simulink model "demonstrator"  (R2021a)
settings: Solver=VariableStepAuto  StartTime=0.0  StopTime=4000/3.2e6  RelTol=1e-3
values from neighbouring files (symbols this model uses):
  f_system = 64e6    (= 64000000)    [setup_demonstrator.m]
  fir_bbuf = reshape([fir_barker_13; fir_barker_13; fir_barker_13], [1, length(fir_barker_13)*3])    [setup_demonstrator.m]
  tx_data = [tx_data mbuf]    [setup_demonstrator.m]
undefined symbols (not defined in the file or in its folder): AXI4, designMultirateFIR, fsystem, Lite, xlfda_numerator
libraries: hdlBasic x533, hdlsllib x35, hdlDSPIP x21, hdlSSR x18, dspmlti4 x14, dspswit3 x8, dspsigops x5, vmcUtilities x4, hdlUtilities x4, simulink x3, dspsigattribs x2, commrandsrc3 x1
(part 4 of 10)

== system demonstrator/Transmitter/AXI-Stream Slave Interface ==
  s_tdata : Inport
  s_tvalid : Inport  Port=2
  s_tlast : Inport  Port=3
  Concat : hdlBasic/Concat  num_inputs=2  XmcBlockStatus=1  maskContainerNames=group1  block_type=concat  block_config=sysgen:Concat_config
  Constant : hdlBasic/Constant  const=0  gui_display_data_type=Fixed-point  arith_type=Unsigned  n_bits=8  bin_pt=0  preci_type=Single  exp_width=8  frac_width=24  explicit_period=off  period=1  XmcBlockStatus=1  maskContainerNames=tabcontainer1  block_type=constant  block_config=sysgen:Constant_config
  Convert : hdlBasic/Convert  gui_display_data_type=Fixed-point  arith_type=Unsigned  n_bits=1  bin_pt=0  float_type=Single  exp_bits=8  fraction_bits=24  quantization=Truncate  overflow=Wrap  en=off  latency=0  pipeline=off  XmcBlockStatus=1  maskContainerNames=group2  block_type=convert  block_config=sysgen:Convert_config
  Down Sample : hdlBasic/Down Sample  sample_ratio=128e6/12.5e3  sample_phase=First Value of Frame  en=off  rst=off  latency=0  XmcBlockStatus=1  maskContainerNames=group1  block_type=dsamp  block_config=sysgen:Downsample_config
  FIFO : hdlBasic/FIFO  mem_type=Block RAM  performance_options=Standard_FIFO  embedded_registers=off  depth=1K  use_asym_data_widths=off  asym_read_width=32  percent_nbits=2  rst=off  rst_latency=2  en=off  use_dcount=off  use_percent_full_port=off  use_almost_empty=off  almost_empty_thresh=2  use_almost_full=off  use_rd_rst_busy=off  use_wr_rst_busy=off  almost_full_thresh=1000  almost_empty_offset=[]  almost_full_offset=[]  explicit_period=off  period=[]  store_only_valid=[]  init_zero=[]  simulation_type=fast_sim  XmcBlockStatus=1  maskContainerNames=tabcontainer1  block_type=fifo  block_config=sysgen:FIFO_config
      settings: infoedit=[]
  Inverter : hdlBasic/Inverter  en=off  latency=0  XmcBlockStatus=1  maskContainerNames=group2  block_type=inv  block_config=sysgen:Inverter_config
  Inverter1 : hdlBasic/Inverter  en=off  latency=0  XmcBlockStatus=1  maskContainerNames=group2  block_type=inv  block_config=sysgen:Inverter_config
  Logical : hdlBasic/Logical  logical_function=AND  inputs=2  en=off  latency=0  precision=Full  arith_type=Unsigned  n_bits=16  bin_pt=0  align_bp=on  overflow=[]  quantization=[]  XmcBlockStatus=1  maskContainerNames=tabcontainer1  block_type=logical  block_config=sysgen:Logical_config
  Mux : hdlBasic/Mux  inputs=2  en=off  latency=0  precision=Full  arith_type=Unsigned  n_bits=16  bin_pt=14  quantization=Truncate  overflow=Wrap  XmcBlockStatus=1  maskContainerNames=tabcontainer1  block_type=mux  block_config=sysgen:Mux_config
  Register : hdlBasic/Register  init=0  rst=off  en=off  XmcBlockStatus=1  maskContainerNames=tabcontainer1  block_type=register  block_config=sysgen:Register_config
  Slice : hdlBasic/Slice  nbits=1  boolean_output=off  mode=Two Bit Locations  bit1=8  base1=LSB of Input  bit0=8  base0=LSB of Input  XmcBlockStatus=1  maskContainerNames=group1  block_type=slice  block_config=sysgen:Slice_config
  Slice1 : hdlBasic/Slice  nbits=1  boolean_output=off  mode=Two Bit Locations  bit1=7  base1=LSB of Input  bit0=0  base0=LSB of Input  XmcBlockStatus=1  maskContainerNames=group1  block_type=slice  block_config=sysgen:Slice_config
  s_axis_tdata : hdlBasic/Gateway In  gui_display_data_type=Fixed-point  arith_type=Unsigned  n_bits=8  bin_pt=0  preci_type=Single  exp_width=8  frac_width=24  rows=1  columns=1  quantization="Round  (unbiased: +/- Inf)"  overflow=Saturate  period=1/128e6  UseAsADC=off  ADCChannel='1'  interface=None  automatic_assignment=on  address_offset=hex2dec('00')  intf_name=''  intf_description=''  default_value=0  timing_constraint=None  locs_specified=off  LOCs={}  io_standard={}  inherit_from_input=off  hdl_port=on  XmcBlockStatus=1  maskContainerNames=group4  block_type=gatewayin  block_config=sysgen:gateway_in_config  block_width_w=590  block_height_w=620  block_width=640  block_height=850
  s_axis_tlast : hdlBasic/Gateway In  gui_display_data_type=Fixed-point  arith_type=Unsigned  n_bits=1  bin_pt=0  preci_type=Single  exp_width=8  frac_width=24  rows=1  columns=1  quantization="Round  (unbiased: +/- Inf)"  overflow=Saturate  period=1/128e6  UseAsADC=off  ADCChannel='1'  interface=None  automatic_assignment=on  address_offset=hex2dec('00')  intf_name=''  intf_description=''  default_value=0  timing_constraint=None  locs_specified=off  LOCs={}  io_standard={}  inherit_from_input=off  hdl_port=on  XmcBlockStatus=1  maskContainerNames=group4  block_type=gatewayin  block_config=sysgen:gateway_in_config  block_width_w=590  block_height_w=620  block_width=640  block_height=850
  s_axis_tready : hdlBasic/Gateway Out  inherit_from_input=on  hdl_port=on  rows=1  columns=1  UseAsDAC=off  DACChannel='1'  interface=None  automatic_assignment=on  address_offset=hex2dec('00')  intf_name=''  intf_description=''  timing_constraint=None  locs_specified=off  LOCs={}  io_standard={}  XmcBlockStatus=1  maskContainerNames=group4  block_type=gatewayout  block_config=sysgen:gateway_out_config  block_width_w=590  block_height_w=620  block_width=620  block_height=750
  s_axis_tvalid : hdlBasic/Gateway In  gui_display_data_type=Boolean  arith_type=Boolean  n_bits=16  bin_pt=14  preci_type=Single  exp_width=8  frac_width=24  rows=1  columns=1  quantization="Round  (unbiased: +/- Inf)"  overflow=Saturate  period=1/128e6  UseAsADC=off  ADCChannel='1'  interface=None  automatic_assignment=on  address_offset=hex2dec('00')  intf_name=''  intf_description=''  default_value=0  timing_constraint=None  locs_specified=off  LOCs={}  io_standard={}  inherit_from_input=off  hdl_port=on  XmcBlockStatus=1  maskContainerNames=group4  block_type=gatewayin  block_config=sysgen:gateway_in_config  block_width_w=590  block_height_w=620  block_width=640  block_height=850
  m_tdata : Outport  VectorParamsAs1DForOutWhenUnconnected=off
  m_tvalid : Outport  Port=2  VectorParamsAs1DForOutWhenUnconnected=off
  m_tlast : Outport  Port=3  VectorParamsAs1DForOutWhenUnconnected=off
  s_tready : Outport  Port=4  VectorParamsAs1DForOutWhenUnconnected=off
  wires:
  s_axis_tready/1 -> s_tready/1
  s_tlast/1 -> s_axis_tlast/1
  s_tvalid/1 -> s_axis_tvalid/1
  s_tdata/1 -> s_axis_tdata/1
  s_axis_tvalid/1 -> FIFO/2
  FIFO/3 -> Inverter/1
  Down Sample/1 -> Inverter1/1
  FIFO/2 -> Down Sample/1
  Register/1 -> Mux/1, Convert/1, m_tvalid/1
  Inverter/1 -> s_axis_tready/1
  Inverter1/1 -> Register/1, FIFO/3
  Logical/1 -> m_tlast/1
  Mux/1 -> m_tdata/1
  FIFO/1 -> Slice/1, Slice1/1
  Constant/1 -> Mux/2
  Convert/1 -> Logical/2
  Slice/1 -> Logical/1
  Concat/1 -> FIFO/1
  s_axis_tdata/1 -> Concat/2
  s_axis_tlast/1 -> Concat/1
  Slice1/1 -> Mux/3

== system demonstrator/Transmitter/Algorithm ==
  note: Serialize data,
      | send (pseudo-random) data from an LFSR if enabled and no input data is present
  note: Encode + pulse shape + interpolate
      | (only I component, Q is fixed at 0)
  enable_data : Inport
  enable_tx : Inport  Port=2
  s_tdata : Inport  Port=3
  s_tvalid : Inport  Port=4
  s_tlast : Inport  Port=5
  BPSK Differential Encoder : Subsystem
  BPSK LFSR : Subsystem
  Gateway Out : hdlBasic/Gateway Out  inherit_from_input=on  hdl_port=off  rows=1  columns=1  UseAsDAC=off  DACChannel='1'  interface=None  automatic_assignment=on  address_offset=hex2dec('00')  intf_name=''  intf_description=''  timing_constraint=None  locs_specified=off  LOCs={}  io_standard={}  XmcBlockStatus=1  maskContainerNames=group4  block_type=gatewayout  block_config=sysgen:gateway_out_config  block_width_w=590  block_height_w=620  block_width=620  block_height=750
  Gateway Out1 : hdlBasic/Gateway Out  inherit_from_input=on  hdl_port=off  rows=1  columns=1  UseAsDAC=off  DACChannel='1'  interface=None  automatic_assignment=on  address_offset=hex2dec('00')  intf_name=''  intf_description=''  timing_constraint=None  locs_specified=off  LOCs={}  io_standard={}  XmcBlockStatus=1  maskContainerNames=group4  block_type=gatewayout  block_config=sysgen:gateway_out_config  block_width_w=590  block_height_w=620  block_width=620  block_height=750
  Gateway Out2 : hdlBasic/Gateway Out  inherit_from_input=on  hdl_port=off  rows=1  columns=1  UseAsDAC=off  DACChannel='1'  interface=None  automatic_assignment=on  address_offset=hex2dec('00')  intf_name=''  intf_description=''  timing_constraint=None  locs_specified=off  LOCs={}  io_standard={}  XmcBlockStatus=1  maskContainerNames=group4  block_type=gatewayout  block_config=sysgen:gateway_out_config  block_width_w=590  block_height_w=620  block_width=620  block_height=750
  Interpolation : Subsystem
  RRC : Subsystem
  TX: Time Domain : Scope  NumInputPorts=3
  Terminator : Terminator
  m_tdata : Outport  VectorParamsAs1DForOutWhenUnconnected=off
  m_tvalid : Outport  Port=2  VectorParamsAs1DForOutWhenUnconnected=off
  wires:
  BPSK LFSR/1(m_tdata) -> BPSK Differential Encoder/2(s_tdata)
  BPSK Differential Encoder/1(m_tdata) -> Gateway Out/1, RRC/1(s_tdata)
  s_tlast/1 -> Terminator/1
  s_tdata/1 -> BPSK LFSR/2(s_tdata)
  s_tvalid/1 -> BPSK LFSR/3(s_tvalid)
  enable_data/1 -> BPSK LFSR/1(enable)
  RRC/1(m_tdata) -> Gateway Out2/1, Interpolation/1(s_tdata)
  Interpolation/2(m_tvalid) -> m_tvalid/1
  Interpolation/1(m_tdata) -> Gateway Out1/1, m_tdata/1
  enable_tx/1 -> BPSK Differential Encoder/1(tx_output)
  Gateway Out/1 -> TX: Time Domain/1
  Gateway Out1/1 -> TX: Time Domain/3
  Gateway Out2/1 -> TX: Time Domain/2

== system demonstrator/Transmitter/Convert Signal ==
  Data In : Inport
  Bit Slice : hdlsllib/Logic and Bit Operations/Bit Slice  lidx=15  ridx=0
      settings: SourceProductBaseCode=SL
  Bit Slice1 : hdlsllib/Logic and Bit Operations/Bit Slice  lidx=31  ridx=16
      settings: SourceProductBaseCode=SL
  Data Type Conversion : DataTypeConversion  OutDataTypeStr=fixdt(1,16,15)  ConvertRealWorld=Stored Integer (SI)
  Data Type Conversion1 : DataTypeConversion  OutDataTypeStr=fixdt(1,16,15)  ConvertRealWorld=Stored Integer (SI)
  Real-Imag to Complex : RealImagToComplex
  Data Out : Outport  VectorParamsAs1DForOutWhenUnconnected=off
  wires:
  Data Type Conversion1/1 -> Real-Imag to Complex/2
  Bit Slice/1 -> Data Type Conversion/1
  Data Type Conversion/1 -> Real-Imag to Complex/1
  Real-Imag to Complex/1 -> Data Out/1
  Data In/1 -> Bit Slice1/1, Bit Slice/1
  Bit Slice1/1 -> Data Type Conversion1/1

== system demonstrator/Transmitter/DMA Read ==
  enable : Inport
  tready : Inport  Port=2
  1-D Lookup Table : Lookup_n-D  NumberOfTableDimensions=1  BreakpointsForDimension1=[0:1:numel(tx_data)-1]  Table=tx_data  TableDataTypeStr=Inherit: Inherit from 'Table data'  ExtrapMethod=Clip  InternalRulePriority=Speed  OutDataTypeStr=Inherit: Inherit from 'Table data'  RndMeth=Simplest  InputSameDT=on
  AND : Logic  IconShape=distinctive  AllPortsSameDT=off  OutDataTypeStr=boolean
  AND1 : Logic  IconShape=distinctive  AllPortsSameDT=off  OutDataTypeStr=boolean
  Compare To Constant : simulink/Logic and Bit Operations/Compare To Constant  relop=>=  const=numel(tx_data)-1  OutDataTypeStr=boolean
  Data Type Conversion : DataTypeConversion  OutDataTypeStr=fixdt(0, ceil(log2(numel(tx_data))), 0)
  HDL Counter : hdlsllib/Sources/HDL Counter  CountType=Free running  CountInit=0  CountStep=1  CountMax=25  CountFromType=Initial value  CountFrom=0  CountResetPort=on  CountLoadPort=off  CountEnbPort=on  CountDirPort=off  CountHitOutputPort=off  CountDataType=Unsigned  CountWordLen=32  CountFracLen=0  CountSampTime=1
  Latch : Subsystem
  Rising Edge Detector : Subsystem
  tdata : Outport  VectorParamsAs1DForOutWhenUnconnected=off
  tvalid : Outport  Port=2  VectorParamsAs1DForOutWhenUnconnected=off
  tlast : Outport  Port=3  VectorParamsAs1DForOutWhenUnconnected=off
  wires:
  1-D Lookup Table/1 -> tdata/1
  Compare To Constant/1 -> AND1/1, HDL Counter/1, Latch/2(R)
  enable/1 -> Rising Edge Detector/1(Input)
  HDL Counter/1 -> Compare To Constant/1, Data Type Conversion/1
  Data Type Conversion/1 -> 1-D Lookup Table/1
  Rising Edge Detector/1(Output) -> Latch/1(S)
  AND/1 -> AND1/2, tvalid/1, HDL Counter/2
  Latch/1(Q) -> AND/2
  tready/1 -> AND/1
  AND1/1 -> tlast/1

== system demonstrator/Transmitter (SIM)/BPSK TX Generation ==
  note: Model DMA (instantiated as BD IP)
  note: Pulse shaping
  note: Input random bits in absence of data
  note: Encode symbols
  note: Scale down amplitude value to correct level
  Enable : Inport
  Bernoulli Binary Generator : commrandsrc3/Bernoulli Binary Generator  ProbabilityOfZero=0.5  SeedSource=Auto  Seed=0  SampleTime=1/100e3  SamplesPerFrame=1  OutputDataType=double  SimulateUsing=Interpreted execution
  CIC Interpolation : dspmlti4/CIC Interpolation  filtFrom=Dialog parameters  filtobj=Hm_interp  ftype=Interpolator  R=320  M=1  N=5  filterInternals=Full precision  BPS=[16 16 16 16]  FLPS=0  outputWordLength=32  outputFracLength=0  launchFVT=off  framing=Allow multirate processing  OutputFrames=off
      settings: SourceProductBaseCode=DS
  Constant : Constant  SampleTime=1/12.5e3
  DBPSK Modulator : Subsystem
  DMA Read : Subsystem
  Data Type Conversion2 : DataTypeConversion  OutDataTypeStr=fixdt(1,16,14)
  FDATool : hdlUtilities/FDATool  block_type=fdatool
      settings: infoedit=FDATool
  FIR Interpolation : dspmlti4/FIR Interpolation  FilterSource=Dialog parameters  PrivateCoeffs=0  h=xlfda_numerator('FDATool')*4  L=4  FilterObject=xlfda_numerator('FDATool')/(max(xlfda_numerator('FDATool')))  framing=Allow multirate processing  outputBufInitCond=0  roundingMode=Floor  overflowMode=off  firstCoeffMode=Binary point scaling  firstCoeffWordLength=16  firstCoeffFracLength=14  firstCoeffDataTypeStr=fixdt(1,16,14)  firstCoeffMin=[]  firstCoeffMax=[]  firstCoeffLastDataTypeStr=fixdt(1,16,14)  outputDataTypeStr=Inherit: Same as accumulator  outputMin=[]  outputMax=[]  outputLastDataTypeStr=Inherit: Same as accumulator
  Multiply : Gain  Gain=fi(0.8192, 1, 16, 14)  ParamDataTypeStr=fixdt(1,16,15)  OutDataTypeStr=fixdt(1,16,14)
  Multiport Switch : MultiPortSwitch  DataPortOrder=Zero-based contiguous  Inputs=2  zeroidx=on
  Shift Arithmetic : ArithShift  BitShiftNumber=33  BitShiftDirection=Right
  TX (SIM): Time Domain : Scope  NumInputPorts=4
  Terminator1 : Terminator
  BPSK : Outport  VectorParamsAs1DForOutWhenUnconnected=off
  wires:
  CIC Interpolation/1 -> TX (SIM): Time Domain/3, Shift Arithmetic/1
  FIR Interpolation/1 -> TX (SIM): Time Domain/2, Data Type Conversion2/1
  Bernoulli Binary Generator/1 -> Multiport Switch/2
  DMA Read/2(tvalid) -> Multiport Switch/1
  DMA Read/1(tdata) -> Multiport Switch/3
  DMA Read/3(tlast) -> Terminator1/1
  Enable/1 -> DMA Read/1(enable)
  Constant/1 -> DMA Read/2(tready)
  Multiport Switch/1 -> DBPSK Modulator/1(Input)
  Multiply/1 -> TX (SIM): Time Domain/4, BPSK/1
  DBPSK Modulator/1(Output) -> TX (SIM): Time Domain/1, FIR Interpolation/1
  Data Type Conversion2/1 -> CIC Interpolation/1
  Shift Arithmetic/1 -> Multiply/1

== system demonstrator/FINNadapter/Decimation/AXI-Stream Master Interface ==
  Re Valid In : Inport
  Re Data In : Inport  Port=2
  Im Valid In : Inport  Port=3
  Im Data In : Inport  Port=4
  Register{,1..3} (4 alike) : hdlBasic/Register  init=0  rst=off  en=off  XmcBlockStatus=1  maskContainerNames=tabcontainer1  block_type=register  block_config=sysgen:Register_config
  m_axis_im_tdata : hdlBasic/Gateway Out  inherit_from_input=off  hdl_port=on  rows=1  columns=1  UseAsDAC=off  DACChannel='1'  interface=None  automatic_assignment=on  address_offset=hex2dec('00')  intf_name=''  intf_description=''  timing_constraint=None  locs_specified=off  LOCs={}  io_standard={}  XmcBlockStatus=1  maskContainerNames=group4  block_type=gatewayout  block_config=sysgen:gateway_out_config  block_width_w=590  block_height_w=620  block_width=620  block_height=750
  m_axis_im_tvalid : hdlBasic/Gateway Out  inherit_from_input=off  hdl_port=on  rows=1  columns=1  UseAsDAC=off  DACChannel='1'  interface=None  automatic_assignment=on  address_offset=hex2dec('00')  intf_name=''  intf_description=''  timing_constraint=None  locs_specified=off  LOCs={}  io_standard={}  XmcBlockStatus=1  maskContainerNames=group4  block_type=gatewayout  block_config=sysgen:gateway_out_config  block_width_w=590  block_height_w=620  block_width=620  block_height=750
  m_axis_re_tdata : hdlBasic/Gateway Out  inherit_from_input=off  hdl_port=on  rows=1  columns=1  UseAsDAC=off  DACChannel='1'  interface=None  automatic_assignment=on  address_offset=hex2dec('00')  intf_name=''  intf_description=''  timing_constraint=None  locs_specified=off  LOCs={}  io_standard={}  XmcBlockStatus=1  maskContainerNames=group4  block_type=gatewayout  block_config=sysgen:gateway_out_config  block_width_w=590  block_height_w=620  block_width=620  block_height=750
  m_axis_re_tvalid : hdlBasic/Gateway Out  inherit_from_input=off  hdl_port=on  rows=1  columns=1  UseAsDAC=off  DACChannel='1'  interface=None  automatic_assignment=on  address_offset=hex2dec('00')  intf_name=''  intf_description=''  timing_constraint=None  locs_specified=off  LOCs={}  io_standard={}  XmcBlockStatus=1  maskContainerNames=group4  block_type=gatewayout  block_config=sysgen:gateway_out_config  block_width_w=590  block_height_w=620  block_width=620  block_height=750
  Re Valid Out : Outport
  Re Data Out : Outport  Port=2
  Im Valid Out : Outport  Port=3
  Im Data Out : Outport  Port=4
  wires:
  Im Data In/1 -> Register3/1
  Re Data In/1 -> Register1/1
  Im Valid In/1 -> Register2/1
  Re Valid In/1 -> Register/1
  m_axis_im_tvalid/1 -> Im Valid Out/1
  m_axis_im_tdata/1 -> Im Data Out/1
  m_axis_re_tvalid/1 -> Re Valid Out/1
  m_axis_re_tdata/1 -> Re Data Out/1
  Register/1 -> m_axis_re_tvalid/1
  Register1/1 -> m_axis_re_tdata/1
  Register2/1 -> m_axis_im_tvalid/1
  Register3/1 -> m_axis_im_tdata/1

== system demonstrator/FINNadapter/Decimation/AXI-Stream Slave Interface ==
  Re Valid In : Inport
  Im Valid In : Inport  Port=2
  Re Data In : Inport  Port=3
  Im Data In : Inport  Port=4
  Constant : hdlBasic/Constant  const=1  gui_display_data_type=Boolean  arith_type=Boolean  n_bits=16  bin_pt=14  preci_type=Single  exp_width=8  frac_width=24  explicit_period=on  period=1/fsystem  XmcBlockStatus=1  maskContainerNames=tabcontainer1  block_type=constant  block_config=sysgen:Constant_config
  Register{,1..3} (4 alike) : hdlBasic/Register  init=0  rst=off  en=off  XmcBlockStatus=1  maskContainerNames=tabcontainer1  block_type=register  block_config=sysgen:Register_config
  Reinterpret : hdlBasic/Reinterpret  force_arith_type=on  arith_type=Unsigned  force_bin_pt=off  bin_pt=0  XmcBlockStatus=1  maskContainerNames=group1  block_type=reinterpret  block_config=sysgen:Reinterpret_config
  Reinterpret1 : hdlBasic/Reinterpret  force_arith_type=on  arith_type=Unsigned  force_bin_pt=off  bin_pt=0  XmcBlockStatus=1  maskContainerNames=group1  block_type=reinterpret  block_config=sysgen:Reinterpret_config
  s_axis_im_tdata : hdlBasic/Gateway In  gui_display_data_type=Fixed-point  arith_type=Signed (2's comp)  n_bits=128  bin_pt=0  preci_type=Single  exp_width=8  frac_width=24  rows=1  columns=1  quantization="Round  (unbiased: +/- Inf)"  overflow=Saturate  period=1/fsystem  UseAsADC=off  ADCChannel='1'  interface=None  automatic_assignment=on  address_offset=hex2dec('00')  intf_name=''  intf_description=''  default_value=0  timing_constraint=None  locs_specified=off  LOCs={}  io_standard={}  inherit_from_input=off  hdl_port=on  XmcBlockStatus=1  maskContainerNames=group4  block_type=gatewayin  block_config=sysgen:gateway_in_config  block_width_w=590  block_height_w=620  block_width=640  block_height=850
  s_axis_im_tready : hdlBasic/Gateway Out  inherit_from_input=off  hdl_port=on  rows=1  columns=1  UseAsDAC=off  DACChannel='1'  interface=None  automatic_assignment=on  address_offset=hex2dec('00')  intf_name=''  intf_description=''  timing_constraint=None  locs_specified=off  LOCs={}  io_standard={}  XmcBlockStatus=1  maskContainerNames=group4  block_type=gatewayout  block_config=sysgen:gateway_out_config  block_width_w=590  block_height_w=620  block_width=620  block_height=750
  s_axis_im_tvalid : hdlBasic/Gateway In  gui_display_data_type=Boolean  arith_type=Boolean  n_bits=16  bin_pt=14  preci_type=Single  exp_width=8  frac_width=24  rows=1  columns=1  quantization="Round  (unbiased: +/- Inf)"  overflow=Saturate  period=1/fsystem  UseAsADC=off  ADCChannel='1'  interface=None  automatic_assignment=on  address_offset=hex2dec('00')  intf_name=''  intf_description=''  default_value=0  timing_constraint=None  locs_specified=off  LOCs={}  io_standard={}  inherit_from_input=off  hdl_port=on  XmcBlockStatus=1  maskContainerNames=group4  block_type=gatewayin  block_config=sysgen:gateway_in_config  block_width_w=590  block_height_w=620  block_width=640  block_height=850
  s_axis_re_tdata : hdlBasic/Gateway In  gui_display_data_type=Fixed-point  arith_type=Signed (2's comp)  n_bits=128  bin_pt=0  preci_type=Single  exp_width=8  frac_width=24  rows=1  columns=1  quantization="Round  (unbiased: +/- Inf)"  overflow=Saturate  period=1/fsystem  UseAsADC=off  ADCChannel='1'  interface=None  automatic_assignment=on  address_offset=hex2dec('00')  intf_name=''  intf_description=''  default_value=0  timing_constraint=None  locs_specified=off  LOCs={}  io_standard={}  inherit_from_input=off  hdl_port=on  XmcBlockStatus=1  maskContainerNames=group4  block_type=gatewayin  block_config=sysgen:gateway_in_config  block_width_w=590  block_height_w=620  block_width=640  block_height=850
  s_axis_re_tready : hdlBasic/Gateway Out  inherit_from_input=off  hdl_port=on  rows=1  columns=1  UseAsDAC=off  DACChannel='1'  interface=None  automatic_assignment=on  address_offset=hex2dec('00')  intf_name=''  intf_description=''  timing_constraint=None  locs_specified=off  LOCs={}  io_standard={}  XmcBlockStatus=1  maskContainerNames=group4  block_type=gatewayout  block_config=sysgen:gateway_out_config  block_width_w=590  block_height_w=620  block_width=620  block_height=750
  s_axis_re_tvalid : hdlBasic/Gateway In  gui_display_data_type=Boolean  arith_type=Boolean  n_bits=16  bin_pt=14  preci_type=Single  exp_width=8  frac_width=24  rows=1  columns=1  quantization="Round  (unbiased: +/- Inf)"  overflow=Saturate  period=1/fsystem  UseAsADC=off  ADCChannel='1'  interface=None  automatic_assignment=on  address_offset=hex2dec('00')  intf_name=''  intf_description=''  default_value=0  timing_constraint=None  locs_specified=off  LOCs={}  io_standard={}  inherit_from_input=off  hdl_port=on  XmcBlockStatus=1  maskContainerNames=group4  block_type=gatewayin  block_config=sysgen:gateway_in_config  block_width_w=590  block_height_w=620  block_width=640  block_height=850
  Re Valid Out : Outport
  Re Data Out : Outport  Port=2
  Im Valid Out : Outport  Port=3
  Im Data Out : Outport  Port=4
  Re Ready Out : Outport  Port=5
  Im Ready Out : Outport  Port=6
  wires:
  s_axis_re_tdata/1 -> Register1/1
  s_axis_im_tdata/1 -> Register/1
  Constant/1 -> s_axis_re_tready/1, s_axis_im_tready/1
  Im Valid In/1 -> s_axis_im_tvalid/1
  s_axis_re_tvalid/1 -> Register3/1
  Register1/1 -> Reinterpret/1
  Register/1 -> Reinterpret1/1
  s_axis_im_tvalid/1 -> Register2/1
  s_axis_im_tready/1 -> Im Ready Out/1
  Re Valid In/1 -> s_axis_re_tvalid/1
  Re Data In/1 -> s_axis_re_tdata/1
  s_axis_re_tready/1 -> Re Ready Out/1
  Im Data In/1 -> s_axis_im_tdata/1
  Register3/1 -> Re Valid Out/1
  Register2/1 -> Im Valid Out/1
  Reinterpret/1 -> Re Data Out/1
  Reinterpret1/1 -> Im Data Out/1

== system demonstrator/FINNadapter/Decimation/Coarse Decimator ==
  Re Valid In : Inport
  Re Data In : Inport  Port=2
  "Im Valid In " : Inport  Port=3
  Im Data In : Inport  Port=4
  Convert : hdlBasic/Convert  gui_display_data_type=Fixed-point  arith_type=Signed (2's comp)  n_bits=16  bin_pt=15  float_type=Single  exp_bits=8  fraction_bits=24  quantization="Round  (unbiased: +/- Inf)"  overflow=Saturate  en=off  latency=0  pipeline=off  XmcBlockStatus=1  maskContainerNames=group2  block_type=convert  block_config=sysgen:Convert_config
  Convert1 : hdlBasic/Convert  gui_display_data_type=Fixed-point  arith_type=Signed (2's comp)  n_bits=16  bin_pt=15  float_type=Single  exp_bits=8  fraction_bits=24  quantization="Round  (unbiased: +/- Inf)"  overflow=Saturate  en=off  latency=0  pipeline=off  XmcBlockStatus=1  maskContainerNames=group2  block_type=convert  block_config=sysgen:Convert_config
  Scalar2Vector : hdlSSR/Scalar2Vector  Commented=through  Width=16  sg_ssr=2  block_type=scalar2vector_ssr  XmcBlockStatus=1  sg_ssr_prev=2  maskContainerNames=group1
  Scalar2Vector1 : hdlSSR/Scalar2Vector  Commented=through  Width=16  sg_ssr=2  block_type=scalar2vector_ssr  XmcBlockStatus=1  sg_ssr_prev=2  maskContainerNames=group1
  Slice : hdlBasic/Slice  Commented=through  nbits=1  boolean_output=off  mode=Two Bit Locations  bit1=31  base1=LSB of Input  bit0=0  base0=LSB of Input  XmcBlockStatus=1  maskContainerNames=group1  block_type=slice  block_config=sysgen:Slice_config
  Slice1 : hdlBasic/Slice  Commented=through  nbits=1  boolean_output=off  mode=Two Bit Locations  bit1=31  base1=LSB of Input  bit0=0  base0=LSB of Input  XmcBlockStatus=1  maskContainerNames=group1  block_type=slice  block_config=sysgen:Slice_config
  Terminator : Terminator
  Terminator2 : Terminator
  Vector Imag FIR 2 : hdlSSR/Vector FIR  coefficientvector=fir2.Numerator  coefficient_sets=1  coefficient_reload=off  filter_type=Decimation  rate_change_type=Integer  interpolation_rate=1  decimation_rate=2  zero_pack_factor=1  sg_ssr=2  coefficient_sign=Signed  quantization=Quantize_Only  coefficient_width=16  bestprecision=on  coefficient_fractional_bits=0  coefficient_structure=Inferred  output_rounding_mode=Full_Precision  output_width=24  filter_architecture=Systolic_Multiply_Accumulate  optimization_goal=Area  optimization_list='None'  data_buffer_type=Automatic  coefficient_buffer_type=Automatic  input_buffer_type=Automatic  output_buffer_type=Automatic  preference_for_other_storage=Automatic  multi_column_support=Automatic  columnconfig='11'  inter_column_pipe_length=4  m_data_has_tready=off  has_aclken=off  has_aresetn=off  reset_data_vector=on  simulation_type=xsim  simulation_model=sysgen:xfirv7_2_cmodel  data_path_portlist={ 's_axis_data_tdata', 'm_axis_data_tdata' }  passband_min=0.0  passband_max=0.5  stopband_min=0.5  stopband_max=1.0  filter_selection=1  gui_behaviour=1  data_sign=Signed  data_width=16  data_fractional_bits=0  data_tuser_width='11'  wrapper_available=true  ip_wrap_arbitrary_binary_point=true  ip_name=FIR Compiler  ip_version=7.2  dsptool_ready=true  ipcore_usecache=true  ipcore_useipmodelcache=true  port_translation_map={ 'aclken' => 'en', 'aresetn' => 'rst' }  run_core_at_system_period=true  ipcore_xco_need_fpga_part=true  ipcore_fpga_part=[]  block_type=fir_compiler_v7_2_ssr  decimation_prev=2  interpolation_prev=1  coeffsets_prev=1  filter_prev=Decimation  channel_sequence=Basic  number_channels=1  pattern_list='P4-0,P4-1,P4-2,P4-3,P4-4'  number_paths=1  data_has_tlast=Not_Required  s_data_has_fifo=off  s_data_has_tuser=Not_Required  m_data_has_tuser=Not_Required  s_config_sync_mode=On_Vector  s_config_method=Single  num_reload_slots=1  XmcBlockStatus=1  sg_ssr_prev=2  maskContainerNames=group10  block_width=657
      settings: block_version=1.0
  Vector Real FIR 2 : hdlSSR/Vector FIR  coefficientvector=fir2.Numerator  coefficient_sets=1  coefficient_reload=off  filter_type=Decimation  rate_change_type=Integer  interpolation_rate=1  decimation_rate=2  zero_pack_factor=1  sg_ssr=2  coefficient_sign=Signed  quantization=Quantize_Only  coefficient_width=16  bestprecision=on  coefficient_fractional_bits=0  coefficient_structure=Inferred  output_rounding_mode=Full_Precision  output_width=24  filter_architecture=Systolic_Multiply_Accumulate  optimization_goal=Area  optimization_list='None'  data_buffer_type=Automatic  coefficient_buffer_type=Automatic  input_buffer_type=Automatic  output_buffer_type=Automatic  preference_for_other_storage=Automatic  multi_column_support=Automatic  columnconfig='11'  inter_column_pipe_length=4  m_data_has_tready=off  has_aclken=off  has_aresetn=off  reset_data_vector=on  simulation_type=xsim  simulation_model=sysgen:xfirv7_2_cmodel  data_path_portlist={ 's_axis_data_tdata', 'm_axis_data_tdata' }  passband_min=0.0  passband_max=0.5  stopband_min=0.5  stopband_max=1.0  filter_selection=1  gui_behaviour=1  data_sign=Signed  data_width=16  data_fractional_bits=0  data_tuser_width='11'  wrapper_available=true  ip_wrap_arbitrary_binary_point=true  ip_name=FIR Compiler  ip_version=7.2  dsptool_ready=true  ipcore_usecache=true  ipcore_useipmodelcache=true  port_translation_map={ 'aclken' => 'en', 'aresetn' => 'rst' }  run_core_at_system_period=true  ipcore_xco_need_fpga_part=true  ipcore_fpga_part=[]  block_type=fir_compiler_v7_2_ssr  decimation_prev=2  interpolation_prev=1  coeffsets_prev=1  filter_prev=Decimation  channel_sequence=Basic  number_channels=1  pattern_list='P4-0,P4-1,P4-2,P4-3,P4-4'  number_paths=1  data_has_tlast=Not_Required  s_data_has_fifo=off  s_data_has_tuser=Not_Required  m_data_has_tuser=Not_Required  s_config_sync_mode=On_Vector  s_config_method=Single  num_reload_slots=1  XmcBlockStatus=1  sg_ssr_prev=2  maskContainerNames=group10  block_width=657
      settings: block_version=1.0
  Vector Reinterpret : hdlSSR/Vector Reinterpret  Commented=through  force_arith_type=on  arith_type="Signed  (2's comp)"  force_bin_pt=on  bin_pt=15  sg_ssr=2  block_type=reinterpret_ssr  XmcBlockStatus=1  sg_ssr_prev=2  maskContainerNames=group1
  Vector Reinterpret1 : hdlSSR/Vector Reinterpret  Commented=through  force_arith_type=on  arith_type="Signed  (2's comp)"  force_bin_pt=on  bin_pt=15  sg_ssr=2  block_type=reinterpret_ssr  XmcBlockStatus=1  sg_ssr_prev=2  maskContainerNames=group1
  Re Valid Out : Outport
  Re Data Out : Outport  Port=2
  Im Valid Out : Outport  Port=3
  Im Data Out : Outport  Port=4
  wires:
  Re Valid In/1 -> Vector Real FIR 2/1
  "Im Valid In "/1 -> Vector Imag FIR 2/1
  Convert/1 -> Im Data Out/1
  Vector Real FIR 2/1 -> Terminator/1
  Vector Imag FIR 2/2 -> Im Valid Out/1
  Vector Real FIR 2/3 -> Convert1/1
  Vector Imag FIR 2/1 -> Terminator2/1
  Re Data In/1 -> Slice/1
  Vector Imag FIR 2/3 -> Convert/1
  Convert1/1 -> Re Data Out/1
  Vector Real FIR 2/2 -> Re Valid Out/1
  Slice/1 -> Scalar2Vector/1
  Vector Reinterpret/1 -> Vector Real FIR 2/2
  Scalar2Vector/1 -> Vector Reinterpret/1
  Scalar2Vector1/1 -> Vector Reinterpret1/1
  Slice1/1 -> Scalar2Vector1/1
  Im Data In/1 -> Slice1/1
  Vector Reinterpret1/1 -> Vector Imag FIR 2/2

== system demonstrator/FINNadapter/Decimation/Convert for Analysis ==
  Valid : Inport
  SSR Real : Inport  Port=2
  SSR Imag : Inport  Port=3
  Data Type Conversion : DataTypeConversion  OutDataTypeStr=fixdt(1,16,15)  ConvertRealWorld=Stored Integer (SI)
  Rate Transition : RateTransition  OutPortSampleTimeOpt=Multiple of input port sample time  OutPortSampleTimeMultiple=2
  Real-Imag to Complex : RealImagToComplex
  SSR to Vector Imag : Subsystem  mask{N=1, w=16, hN=1, hw=16}
      mask prompts: N "Samples per clock cycle:"; w "Wordlength:"
      mask init:
      | if ~isequal(get_param(gcb, 'N'), get_param(gcb, 'hN')) ||...
      |         ~isequal(get_param(gcb, 'w'), get_param(gcb, 'hw'))
      |     % Delete all blocks except input and output ports
      |     delete_block(setxor(setdiff(...
      |         find_system(gcb,'LookUnderMasks','on'),...
      |         {[gcb, '/Vector'], [gcb, '/SSR']}), gcb));
      | 
      |     % Delete all wires
      |     delete_line(find_system(gcb, 'FindAll', 'on', 'LookUnderMasks',...
      |         'on', 'SearchDepth', 3, 'Type', 'line', 'Connected', 'off'));
      | 
      |     % Add the matrix concatenation block
      |     add_block('hdlsllib/Math Operations/Matrix Concatenate',...
      |         [gcb, '/Matrix Concatenate'],...
      |         'Position', [155 55 205 330]);
      |     set_param([gcb, '/Matrix Concatenate'], 'NumInputs', num2str(N));
      |     set_param([gcb, '/Matrix Concatenate'], 'ConcatenateDimension', num2str(1));
      |     
      |     % Add wire to output
      |     add_line(gcb, 'Matrix Concatenate/1', 'Vector/1');
      | 
      |     % Add slice blocks and connect wires
      |     for i = 0:N-1
      |         add_block('hdlsllib/Logic and Bit Operations/Bit Slice',...
      |             [gcb, '/Bit Slice', num2str(i)],...
      |             'Position', [0 82+i*90 45 128+i*90]);
      |         set_param([gcb, '/Bit Slice', num2str(i)], 'ridx', num2str(0+i*(w)));
      |         set_param([gcb, '/Bit Slice', num2str(i)], 'lidx', num2str((w-1)+i*(w)));
      |         add_line(gcb, 'SSR/1', ['Bit Slice', num2str(i), '/1'],...
      |             'autorouting', 'on');
      |         add_line(gcb, ['Bit Slice', num2str(i), '/1'],...
      |             ['Matrix Concatenate/', num2str(i+1)],...
      |             'autorouting', 'on');
      |     end
      |     
      |     % Set the hidden attribute to prevent unnecessary changes in
      |     % architecture while generating HDL Code.
      |     set_param(gcb, 'hN', get_param(gcb, 'N'));
      |     set_param(gcb, 'hw', get_param(gcb, 'w'));
      | end
      mask DialogControl DescGroupVar Prompt: SSR to Vector
      mask DialogControl DescTextVar Prompt: Convert the SSR vector format based on the wordlength and expected number of samples per clock cycle.
  SSR to Vector Real : Subsystem  mask{N=1, w=16, hN=1, hw=16}
      mask prompts: N "Samples per clock cycle:"; w "Wordlength:"
      mask init: same as demonstrator/FINNadapter/Decimation/Convert for Analysis/SSR to Vector Imag
      mask DialogControl DescGroupVar Prompt: SSR to Vector
      mask DialogControl DescTextVar Prompt: Convert the SSR vector format based on the wordlength and expected number of samples per clock cycle.
  Terminator : Terminator
  Data : Outport
  wires:
  SSR to Vector Imag/1(Vector) -> Real-Imag to Complex/2
  SSR to Vector Real/1(Vector) -> Real-Imag to Complex/1
  SSR Real/1 -> SSR to Vector Real/1(SSR)
  Rate Transition/1 -> Data Type Conversion/1
  Real-Imag to Complex/1 -> Rate Transition/1
  SSR Imag/1 -> SSR to Vector Imag/1(SSR)
  Data Type Conversion/1 -> Data/1
  Valid/1 -> Terminator/1

== system demonstrator/FINNadapter/Decimation/Fine Decimator ==
  Re Valid In : Inport
  Re Data In : Inport  Port=2
  Im Valid In : Inport  Port=3
  Im Data In : Inport  Port=4
  Decimation : Inport  Port=5
  Decimators : Subsystem
  Switch : Subsystem
      settings: PortSchema="{\"entries\":[{\"content\":{\"sides\":[{\"content\":{\"connectorIds\":[\"In1\",\"In2\",\"In3\",\"In4\",\"In5\",\"In6\",\"In7\",\"In8\",\"In9\",\"In10\",\"In11\",\"In12\",\"In13\",\"In14\",\"In15\",\"In16\",\"In17\",\"In18\",\"In19\",\"In20\",\"In21\",\"In22\",\"In23\",\"In24\",\"In25\",\"In26\",\"In27\",\"In28\",\"In29\",\"In30\",\"In31\",\"In32\"]},\"type\":\"ConnectorPlacement.EquallySpacedRectSide\",\"uuid\":\"774f33ce-0ead-458b-bf10-c8d40cb77827\"},{\"content\":{\"connectorIds\":[\"Out1\",\"Out2\",\"Out3\",\"Out4\"],\"side\":\"RIGHT\"},\"type\":\"ConnectorPlacement.EquallySpacedRectSide\",\"uuid\":\"3161ebc9-56ab-443f-932f-613d597be8f5\"},{\"content\":{\"connectorIds\":[\"In33\"],\"side\":\"TOP\"},\"type\":\"ConnectorPlacement.EquallySpacedRectSide\",\"uuid\":\"93ea1115-8d53-4d81-a694-b06c3ff8ec0e\"}]},\"type\":\"ConnectorPlacement.EquallySpacedConnector\",\"uuid\":\"a015abf8-23b8-43ad-942c-35dd9b4ce6a7\"}],\"packageUris\":[\"http://schema.mathworks.com/mf0/Connector/19700101\"],\"version\":\"1.0\"}"
  Re Valid Out : Outport
  Re Data Out : Outport  Port=2
  Im Valid Out : Outport  Port=3
  Im Data Out : Outport  Port=4
  wires:
  Switch/2(Re Data Out) -> Re Data Out/1
  Switch/1(Re Valid Out) -> Re Valid Out/1
  Switch/4(Im Data Out) -> Im Data Out/1
  Re Data In/1 -> Decimators/2(Re Data In)
  Re Valid In/1 -> Decimators/1(Re Valid In)
  Im Valid In/1 -> Decimators/3("Im Valid In ")
  Im Data In/1 -> Decimators/4(Im Data In)
  Decimation/1 -> Switch/33(Sel)
  Switch/3(Im Valid Out) -> Im Valid Out/1
  Decimators/2(Re Valid 1) -> Switch/2(Re Valid 1)
  Decimators/3(Re Valid 2) -> Switch/3(Re Valid 2)
  Decimators/4(Re Valid 3) -> Switch/4(Re Valid 3)
  Decimators/5(Re Valid 4) -> Switch/5(Re Valid 4)
  Decimators/6(Re Valid 5) -> Switch/6(Re Valid 5)
  Decimators/7(Re Valid 6) -> Switch/7(Re Valid 6)
  Decimators/10(Re Data 1) -> Switch/10(Re Data 1)
  Decimators/11(Re Data 2) -> Switch/11(Re Data 2)
  Decimators/12(Re Data 3) -> Switch/12(Re Data 3)
  Decimators/13(Re Data 4) -> Switch/13(Re Data 4)
  Decimators/14(Re Data 5) -> Switch/14(Re Data 5)
  Decimators/15(Re Data 6) -> Switch/15(Re Data 6)
  Decimators/18(Im Valid 1) -> Switch/18(Im Valid 1)
  Decimators/19(Im Valid 2) -> Switch/19(Im Valid 2)
  Decimators/20(Im Valid 3) -> Switch/20(Im Valid 3)
  Decimators/21(Im Valid 4) -> Switch/21(Im Valid 4)
  Decimators/22(Im Valid 5) -> Switch/22(Im Valid 5)
  Decimators/23(Im Valid 6) -> Switch/23(Im Valid 6)
  Decimators/26(Im Data 1) -> Switch/26(Im Data 1)
  Decimators/27(Im Data 2) -> Switch/27(Im Data 2)
  Decimators/28(Im Data 3) -> Switch/28(Im Data 3)
  Decimators/29(Im Data 4) -> Switch/29(Im Data 4)
  Decimators/30(Im Data 5) -> Switch/30(Im Data 5)
  Decimators/31(Im Data 6) -> Switch/31(Im Data 6)
  Decimators/1(Re Valid 0) -> Switch/1(Re Valid 0)
  Decimators/9(Re Data 0) -> Switch/9(Re Data 0)
  Decimators/17(Im Valid 0) -> Switch/17(Im Valid 0)
  Decimators/25(Im Data 0) -> Switch/25(Im Data 0)
  Decimators/8(Re Valid 7) -> Switch/8(Re Valid 7)
  Decimators/16(Re Data 7) -> Switch/16(Re Data 7)
  Decimators/24(Im Valid 7) -> Switch/24(Im Valid 7)
  Decimators/32(Im Data 7) -> Switch/32(Im Data 7)

== system demonstrator/FINNadapter/Decimation/SSR Switch ==
  Re Valid In : Inport
  Re Data In : Inport  Port=2
  "Im Valid In " : Inport  Port=3
  Im Data In : Inport  Port=4
  SSR Re Valid In : Inport  Port=5
  SSR Re Data In : Inport  Port=6
  SSR Im Valid In : Inport  Port=7
  SSR Im Data In : Inport  Port=8
  Decimation : Inport  Port=9
  Mux{,1..3} (4 alike) : hdlBasic/Mux  inputs=2  en=off  latency=1  precision=Full  arith_type=Unsigned  n_bits=16  bin_pt=14  quantization=Truncate  overflow=Wrap  XmcBlockStatus=1  maskContainerNames=tabcontainer1  block_type=mux  block_config=sysgen:Mux_config
  Re Valid Out : Outport
  Re Data Out : Outport  Port=2
  Im Valid Out : Outport  Port=3
  Im Data Out : Outport  Port=4
  wires:
  SSR Re Valid In/1 -> Mux/2
  SSR Im Valid In/1 -> Mux2/2
  SSR Im Data In/1 -> Mux3/2
  SSR Re Data In/1 -> Mux1/2
  Re Valid In/1 -> Mux/3
  Re Data In/1 -> Mux1/3
  Im Data In/1 -> Mux3/3
  "Im Valid In "/1 -> Mux2/3
  Mux3/1 -> Im Data Out/1
  Mux2/1 -> Im Valid Out/1
  Mux1/1 -> Re Data Out/1
  Decimation/1 -> Mux2/1, Mux3/1, Mux1/1, Mux/1
  Mux/1 -> Re Valid Out/1

== system demonstrator/FINNadapter/Decimation/Scalar Converter ==
  Re Valid In : Inport
  Re Data In : Inport  Port=2
  "Im Valid In " : Inport  Port=3
  Im Data In : Inport  Port=4
  Concat : hdlBasic/Concat  num_inputs=2  XmcBlockStatus=1  maskContainerNames=group1  block_type=concat  block_config=sysgen:Concat_config
  Concat1 : hdlBasic/Concat  num_inputs=2  XmcBlockStatus=1  maskContainerNames=group1  block_type=concat  block_config=sysgen:Concat_config
  Constant : hdlBasic/Constant  const=0  gui_display_data_type=Fixed-point  arith_type=Unsigned  n_bits=112  bin_pt=0  preci_type=Single  exp_width=8  frac_width=24  explicit_period=on  period=1/64e6  XmcBlockStatus=1  maskContainerNames=tabcontainer1  block_type=constant  block_config=sysgen:Constant_config
  Reinterpret : hdlBasic/Reinterpret  force_arith_type=on  arith_type=Unsigned  force_bin_pt=on  bin_pt=0  XmcBlockStatus=1  maskContainerNames=group1  block_type=reinterpret  block_config=sysgen:Reinterpret_config
  Reinterpret1 : hdlBasic/Reinterpret  force_arith_type=on  arith_type=Unsigned  force_bin_pt=on  bin_pt=0  XmcBlockStatus=1  maskContainerNames=group1  block_type=reinterpret  block_config=sysgen:Reinterpret_config
  Re Valid Out : Outport
  Re Data Out : Outport  Port=2
  Im Valid Out : Outport  Port=3
  Im Data Out : Outport  Port=4
  wires:
  Concat1/1 -> Im Data Out/1
  Concat/1 -> Re Data Out/1
  Reinterpret1/1 -> Concat1/2
  Reinterpret/1 -> Concat/2
  "Im Valid In "/1 -> Im Valid Out/1
  Re Valid In/1 -> Re Valid Out/1
  Im Data In/1 -> Reinterpret1/1
  Constant/1 -> Concat/1, Concat1/1
  Re Data In/1 -> Reinterpret/1

== system demonstrator/FINNadapter/Decimation/Stimulus and Channel ==
  Channel : Subsystem
  Data Type Conversion1 : DataTypeConversion  OutDataTypeStr=fixdt(0,128,0)  ConvertRealWorld=Stored Integer (SI)
  Data Type Conversion2 : DataTypeConversion  OutDataTypeStr=fixdt(0,128,0)  ConvertRealWorld=Stored Integer (SI)
  Enable : Constant  OutDataTypeStr=boolean  SampleTime=-1
  Transmitter : Subsystem  TreatAsAtomicUnit=on
  Value : Constant  Value=hex2dec('7FFF7FFF')  OutDataTypeStr=uint32  SampleTime=-1
  Valid Real : Outport
  Valid Imag : Outport  Port=2
  Data Real : Outport  Port=3
  Data Imag : Outport  Port=4
  wires:
  Channel/1(Valid Real) -> Valid Real/1
  Channel/3(Valid Imag) -> Valid Imag/1
  Value/1 -> Transmitter/2(Value)  "Value"
  Transmitter/2(Data) -> Channel/2(Data)
  Transmitter/1(Valid) -> Channel/1(Valid)
  Enable/1 -> Transmitter/1(Enable)  "Enable"
  Data Type Conversion1/1 -> Data Real/1
  Channel/2(Data Real) -> Data Type Conversion1/1
  Channel/4(Data Imag) -> Data Type Conversion2/1
  Data Type Conversion2/1 -> Data Imag/1

== system demonstrator/Inspector/Data Inspector Module/Data Inspector Core ==
  packet_size : Inport
  tvalid_in : Inport  Port=2
  tdata_in : Inport  Port=3
  enable : Inport  Port=4
  reset : Inport  Port=5
  Master AXI-Stream Interface : Subsystem
  Simple Slave AXI-Stream Interface : Subsystem
  tvalid_out : Outport  VectorParamsAs1DForOutWhenUnconnected=off
  tdata_out : Outport  Port=2  VectorParamsAs1DForOutWhenUnconnected=off
  tlast_out : Outport  Port=3  VectorParamsAs1DForOutWhenUnconnected=off
  wires:
  Master AXI-Stream Interface/2(tdata_out) -> tdata_out/1
  Master AXI-Stream Interface/3(tlast_out) -> tlast_out/1
  Master AXI-Stream Interface/1(tvalid_out) -> tvalid_out/1
  tvalid_in/1 -> Simple Slave AXI-Stream Interface/1(tvalid_in)
  tdata_in/1 -> Simple Slave AXI-Stream Interface/2(tdata_in)
  enable/1 -> Master AXI-Stream Interface/3(enable)
  packet_size/1 -> Master AXI-Stream Interface/5(packetsize)
  Simple Slave AXI-Stream Interface/1(tvalid_out) -> Master AXI-Stream Interface/1(tvalid_in)
  Simple Slave AXI-Stream Interface/2(tdata_out) -> Master AXI-Stream Interface/2(tdata_in)
  reset/1 -> Master AXI-Stream Interface/4(reset)

== system demonstrator/Inspector/s00_axis/Enabled Counter ==
  Counter Limited : simulink/Sources/Counter Limited  uplimit=127  tsamp=1/(400e3)
  Count : Outport  VectorParamsAs1DForOutWhenUnconnected=off
  wires:
  Counter Limited/1 -> Count/1

== system demonstrator/RF-ADC/NCO and Mixer/RF-ADC Coarse Mixer ==
  Data In : Inport
  Constant : Constant  Value=mc  OutDataTypeStr=fixdt(0,2,0)  SampleTime=-1
  Data Type Conversion : DataTypeConversion  OutDataTypeStr=fixdt(1,16,14)
  Multiport Switch1 : MultiPortSwitch  DataPortOrder=Zero-based contiguous  zeroidx=on
  Negate : Subsystem
  fs_2 : Subsystem
  fs_4 : Subsystem
  Data Out : Outport  VectorParamsAs1DForOutWhenUnconnected=off
  wires:
  Multiport Switch1/1 -> Data Type Conversion/1
  fs_2/1(Data Out) -> Multiport Switch1/2
  Constant/1 -> Multiport Switch1/1
  Data In/1 -> fs_4/1(Data In), fs_2/1(Data In)
  Negate/1(Data Out) -> Multiport Switch1/4
  fs_4/1(Data Out) -> Negate/1(Data In), Multiport Switch1/3
  Data Type Conversion/1 -> Data Out/1

== system demonstrator/RF-ADC/NCO and Mixer/RF-ADC Fine Mixer ==
  Data In : Inport
  Complex to Real-Imag : ComplexToRealImag
  Constant : Constant  Value=0  SampleTime=-1
  Multiport Switch : MultiPortSwitch  DataPortOrder=Zero-based contiguous  Inputs=2  zeroidx=on
  NCO : dspsigops/NCO  AccIncSrc=Specify via dialog  AccInc=fix((((fc*1e9)*(2^18))/(fs))*2^30)  PhaseOffsetSrc=Specify via dialog  PhaseOffset=fix((((2^18)*fph)/(2*pi))*2^30)  AccumWL=48  HasDither=off  DitherWL=4  PNgeneratorLength=19  HasPhaseQuantizer=on  TableDepth=18  HasOutputPhaseError=off  Formula=Sine and cosine  DataType=Binary point scaling  OutputWL=16  OutputFL=14  CompMethod=Table lookup (no interpolation)  SampleTime=1/(fs)  SamplesPerFrame=ssr  OutputFrames=off
      settings: SourceProductBaseCode=DS
  Product : Product  OutDataTypeStr=fixdt(1,16,14)
  Product1 : Product  OutDataTypeStr=fixdt(1,16,14)
  Real-Imag to Complex : RealImagToComplex
  Real-Imag to Complex1 : RealImagToComplex
  Shift Arithmetic : ArithShift  BitShiftNumber=1  BitShiftDirection=Right
  Shift Arithmetic1 : ArithShift  BitShiftNumber=1  BitShiftDirection=Right
  Data Out : Outport  VectorParamsAs1DForOutWhenUnconnected=off
  wires:
  Data In/1 -> Product1/1, Product/1
  Constant/1 -> Multiport Switch/1
  Multiport Switch/1 -> Data Out/1
  Complex to Real-Imag/2 -> Shift Arithmetic/1
  Complex to Real-Imag/1 -> Shift Arithmetic1/1
  Shift Arithmetic1/1 -> Real-Imag to Complex1/1
  Shift Arithmetic/1 -> Real-Imag to Complex1/2
  Real-Imag to Complex1/1 -> Multiport Switch/3
  NCO/1 -> Product/2
  NCO/2 -> Product1/2
  Real-Imag to Complex/1 -> Multiport Switch/2, Complex to Real-Imag/1
  Product1/1 -> Real-Imag to Complex/1
  Product/1 -> Real-Imag to Complex/2

== system demonstrator/RF-DAC/NCO and Mixer/RF-DAC Coarse Mixer ==
  Data In : Inport
  Add2 : Sum
  Complex to Real-Imag : ComplexToRealImag
  Constant : Constant  Value=mc  OutDataTypeStr=fixdt(0,2,0)  SampleTime=-1
  Multiport Switch1 : MultiPortSwitch  DataPortOrder=Zero-based contiguous  zeroidx=on
  Negate : Subsystem
  fs_2 : Subsystem
  fs_4 : Subsystem
  Data Out : Outport  VectorParamsAs1DForOutWhenUnconnected=off
  wires:
  fs_4/1(Data Out) -> Multiport Switch1/3, Negate/1(Data In)
  Negate/1(Data Out) -> Multiport Switch1/4
  Data In/1 -> fs_2/1(Data In), fs_4/1(Data In)
  Constant/1 -> Multiport Switch1/1
  fs_2/1(Data Out) -> Multiport Switch1/2
  Multiport Switch1/1 -> Complex to Real-Imag/1
  Complex to Real-Imag/1 -> Add2/1
  Complex to Real-Imag/2 -> Add2/2
  Add2/1 -> Data Out/1

== system demonstrator/RF-DAC/NCO and Mixer/RF-DAC Fine Mixer ==
  Data In : Inport
  Add2 : Sum
  Complex to Real-Imag1 : ComplexToRealImag
  Constant : Constant  Value=0  OutDataTypeStr=boolean  SampleTime=-1
  Multiport Switch : MultiPortSwitch  DataPortOrder=Zero-based contiguous  Inputs=2  zeroidx=on
  NCO : dspsigops/NCO  AccIncSrc=Specify via dialog  AccInc=fix((((fc*1e9)*(2^18))/(fs))*2^30)  PhaseOffsetSrc=Specify via dialog  PhaseOffset=fix((((2^18)*fph)/(2*pi))*2^30)  AccumWL=48  HasDither=off  DitherWL=4  PNgeneratorLength=19  HasPhaseQuantizer=on  TableDepth=18  HasOutputPhaseError=off  Formula=Sine and cosine  DataType=Binary point scaling  OutputWL=16  OutputFL=14  CompMethod=Table lookup (no interpolation)  SampleTime=1/(fs)  SamplesPerFrame=ssr  OutputFrames=off
      settings: SourceProductBaseCode=DS
  Product1 : Product  OutDataTypeStr=Inherit: Same as first input
  Product4 : Product  OutDataTypeStr=Inherit: Same as first input
  Shift Arithmetic1 : ArithShift  BitShiftNumber=1  BitShiftDirection=Right
  Data Out : Outport  VectorParamsAs1DForOutWhenUnconnected=off
  wires:
  Shift Arithmetic1/1 -> Multiport Switch/3
  Add2/1 -> Multiport Switch/2, Shift Arithmetic1/1
  Multiport Switch/1 -> Data Out/1
  Constant/1 -> Multiport Switch/1
  Data In/1 -> Complex to Real-Imag1/1
  Product4/1 -> Add2/1
  NCO/1 -> Product4/2
  NCO/2 -> Product1/1
  Complex to Real-Imag1/1 -> Product1/2
  Complex to Real-Imag1/2 -> Product4/1
  Product1/1 -> Add2/2
